simulink model "wheel_leg_backup_621"  (R2025b)
settings: Solver=VariableStepAuto  StartTime=0.0  StopTime=10  FixedStep=0.0001  RelTol=1e-3
undefined symbols (not defined in the file): g, M_L_support, X, Y, Z
libraries: sm_lib x76, nesl_utility x14, slpidlib x1
(part 3 of 3)

== matlab function wheel_leg_backup_621/MATLAB Function1 ==
  data: L0 input; K output
function K = simcall_get_k_cubic_length(L0)

K = zeros(2,6);              % 明确告诉 Simulink：K 是 2×6
K(:,:) = get_k_cubic_length(L0);

end

== matlab function wheel_leg_backup_621/MATLAB Function ==
  data: pai1 input; L0 output; pai0 output; pai4 input
function [L0,pai0] = simcall_fivebar_kinematics_func(pai1,pai4)

[L0,pai0] = fivebar_kinematics_func(pai1,pai4);

== matlab function wheel_leg_backup_621/MATLAB Function2 ==
  data: K input; theta input; T output; dtheta input; x input; Tp output; dx input; phi input; dphi input; theta_d input; dtheta_d input; x_d input; dx_d input; phi_d input; dphi_d input
function [T,Tp] = Get_U(K, theta, dtheta, x, dx, phi, dphi, ...
                                          theta_d, dtheta_d, x_d, dx_d, phi_d, dphi_d)
   
    X = [
        theta;
        dtheta;
        x;
        dx;
        phi;
        dphi
    ];
    
    Xd = [
        theta_d;
        dtheta_d;
        x_d;
        dx_d;
        phi_d;
        dphi_d
    ];
    U = -K*(X - Xd);
    T = U(1);
    Tp = U(2);
end

== matlab function wheel_leg_backup_621/MATLAB Function3 ==
  data: phi1 input; dL0 output; phi4 input; dphi1 input; dphi4 input; dphi0 output
function [dL0,dphi0] = simcall_fivebar_velocity_func(phi1,phi4,dphi1,dphi4)

[dL0,dphi0] = fivebar_velocity_func(phi1,phi4,dphi1,dphi4);

end

== matlab function wheel_leg_backup_621/MATLAB Function4 ==
  data: phi0 input; theta output; dphi0 input; body_phi input; body_dphi input; dtheta output
function [theta,dtheta] = simcall_fivebar_theta_func(phi0,dphi0,body_phi,body_dphi)

    [theta,dtheta] = fivebar_theta_func(phi0,dphi0,body_phi,body_dphi);

end

== matlab function wheel_leg_backup_621/MATLAB Function5 ==
  data: phi1 input; T1 output; phi4 input; F_command input; Tp input; T4 output
function [T1,T4] = simcall_fivebar_vmc_torque_func(phi1,phi4,F_command,Tp)

    [T1,T4] = fivebar_vmc_torque_func(phi1,phi4,F_command,Tp);
    
end
